simulink model "PubIfDecisionLM_MDL"  (R2020b)
settings: configuration reference "DspaceConfig" (kept outside this file)
PostLoadFcn:
  | if any(exist('dsrtsu_mdlpostloadfcn', 'file') ~= 0), dsrtsu_mdlpostloadfcn('Execute', bdroot); end
InitFcn:
  | , if any(exist('dsmpb_private', 'file') ~= 0), dsmpb_private('dsmpb_mdlclblib', 'Init', bdroot); end,
undefined symbols (not defined in the file or in its folder): OFM_OBJ_FUSIONTYPE_E, OFM_OBJ_MOVINGSTATE_E, OFM_OBJ_ORIENTATION_E, OFM_OBJ_TYPE_E, P_LM_Cyc, P_LM_EMLHistKapRcdBufSize, P_LM_EMLHistTrajBaseDis, P_LM_EMLHistTrajPNum, P_LM_EMLKapCorrMaxThre, P_LM_EMLMinKapThre, P_LM_EMLPathDisDiffThre, P_LM_EMLQuaFiltPar, P_LM_EMLTurnActKapThre, P_LM_EMLValidQuaThre, P_LM_FntPath1Disgap, P_LM_FntPath1MinDis, P_LM_FntPath1Timegap, P_LM_FntPath2Disgap, P_LM_FntPath2MinDis, P_LM_FntPath2Timegap, P_LM_FntPath3Disgap, P_LM_FntPath3MinDis, P_LM_FntPath3Timegap, P_LM_FusBLParFiltP, P_LM_FusEVDifC2Thre, P_LM_FusEVOPath1AllVSLDisThre, P_LM_FusEVOPath1AllVSLLostNumThre, P_LM_FusEVOPath1AllVSLQuaThre, P_LM_FusEVOPath1OTLFacNLC, P_LM_FusOTLQuaThre, P_LM_FusOTLSW, P_LM_FusParC0Index, P_LM_FusParC1Index, P_LM_FusParC2Index, P_LM_FusParC3Index, P_LM_FusVSLQuaThre, P_LM_FusVSLSW, P_LM_FusVSLValidSteerWheerAngThre, P_LM_FusVSLValidVxvThre, P_LM_LaneWidth, P_LM_OTLBufTPInfoEvaFactor, P_LM_OTLObjNum, P_LM_OTLObjSelectAgeThre, P_LM_OTLObjSelectDxAssessVx, P_LM_OTLObjSelectDxThre, P_LM_OTLObjSelectVxThre, P_LM_OTLObjSelectVyAssessDx, P_LM_OTLObjSelectVyThre, P_LM_OTLTrajPntBaseDis, P_LM_OTLTrajStdThre, P_LM_VSLAvailLineNum, P_LM_VSLBLSDiffThre, P_LM_VSLBLSDisRatio, P_LM_VSLFusBLParFiltP_C1, P_LM_VSLFusBLParFiltP_C2, P_LM_VSLFusBLParFiltP_C3, P_LM_VSLFusBLParFiltP_Quality, P_LM_VSLHistTrajBaseDis, P_LM_VSLHistTrajPNum, P_LM_VSLLCC0diff ... (+18)
libraries: simulink x145, LM_LIB x43
(part 1 of 24)
PreSaveFcn:
  | , if any(exist('dsmpb_private', 'file') ~= 0), dsmpb_private('dsmpb_mdlclblib', 'PreSave', bdroot); end,
CloseFcn:
  | , if any(exist('dsmpb_private', 'file') ~= 0), dsmpb_private('dsmpb_mdlclblib', 'Close', bdroot); end,
settings Model: DataDictionary=HWA_DDs.sldd  RTICANMMDATA=struct('GeneralSetupData',struct('modelroot','C:\Users\GW00133806\Desktop\ADAS_Store\Project\V61_Autobox_Noa\LM_TOS','generalsettings',struct('filesettings',struct('destfolder',struct('Name','RTICANMM_FILES','Check',1),'buildfolder',struct('Name','.','Check',1),'AbsDestfolder',struct('Name','C:\Users\GW00133806\Desktop\ADAS_Store\Project\V61_Autobox_Noa\LM_TOS\RTICANMM_FILES'),'AbsBuildfolder',struct('Name','C:\Users\GW00133806\Desktop\ADAS_Store\Project\V61_Autobox_Noa\LM_TOS'))),'options',struct('addpaths',1,'rmpaths',1,'addtrcexclusion',false,'cannavigator',struct('checkmonitoring',0),'show_usrtrc',0,'use_usrtrc',0),'advanced',struct('options',ones(1,100)),'MPSetup',{{}},'RTI',struct('Type','DSRT','Ver','4.2','Date','02-Nov-2019'),'modelname','PubIfDecisionLM_MDL','block','PubIfDecisionLM_MDL'))  DSRTSU_INTERNAL_RTIFPGA=150  Creator=GW00180895  LastModifiedBy=GW00133806
settings ConfigSetRef: SourceName=DspaceConfig

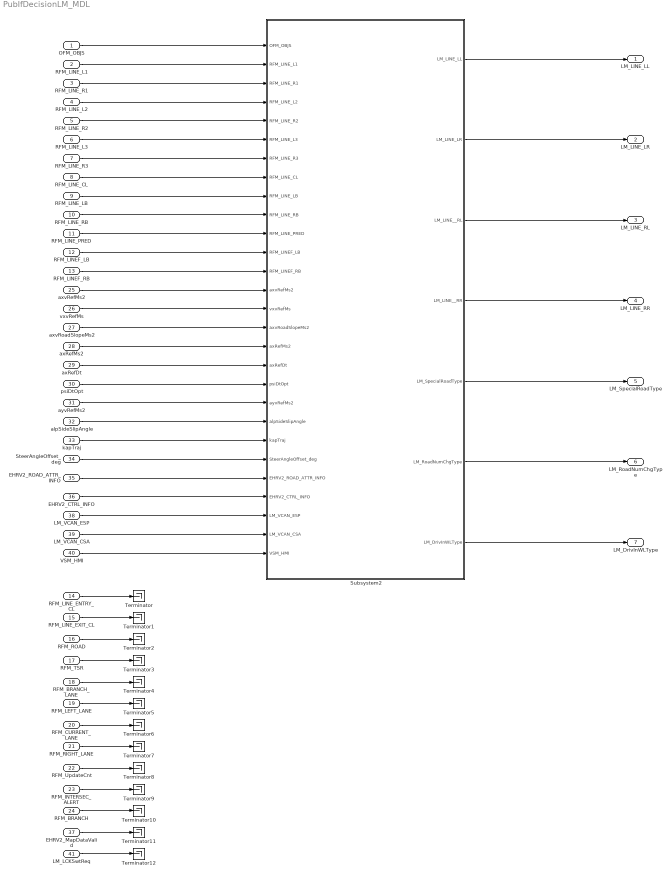
== system PubIfDecisionLM_MDL ==
  OFM_OBJS : Inport  OutDataTypeStr=Bus: OFM_OBJ_BUS  PortDimensions=1  BusOutputAsStruct=on
  RFM_LINE_L1 : Inport  Port=2  OutDataTypeStr=Bus: RFM_LINE_BUS  PortDimensions=1  BusOutputAsStruct=on
  RFM_LINE_R1 : Inport  Port=3  OutDataTypeStr=Bus: RFM_LINE_BUS  PortDimensions=1  BusOutputAsStruct=on
  RFM_LINE_L2 : Inport  Port=4  OutDataTypeStr=Bus: RFM_LINE_BUS  PortDimensions=1  BusOutputAsStruct=on
  RFM_LINE_R2 : Inport  Port=5  OutDataTypeStr=Bus: RFM_LINE_BUS  PortDimensions=1  BusOutputAsStruct=on
  RFM_LINE_L3 : Inport  Port=6  OutDataTypeStr=Bus: RFM_LINE_BUS  PortDimensions=1  BusOutputAsStruct=on
  RFM_LINE_R3 : Inport  Port=7  OutDataTypeStr=Bus: RFM_LINE_BUS  PortDimensions=1  BusOutputAsStruct=on
  RFM_LINE_CL : Inport  Port=8  OutDataTypeStr=Bus: RFM_LINE_BUS  PortDimensions=1  BusOutputAsStruct=on
  RFM_LINE_LB : Inport  Port=9  OutDataTypeStr=Bus: RFM_LINE_BUS  PortDimensions=1  BusOutputAsStruct=on
  RFM_LINE_RB : Inport  Port=10  OutDataTypeStr=Bus: RFM_LINE_BUS  PortDimensions=1  BusOutputAsStruct=on
  RFM_LINE_PRED : Inport  Port=11  OutDataTypeStr=Bus: RFM_LINE_BUS  PortDimensions=1  BusOutputAsStruct=on
  RFM_LINEF_LB : Inport  Port=12  OutDataTypeStr=Bus: RFM_LINE_BUS  PortDimensions=1  BusOutputAsStruct=on
  RFM_LINEF_RB : Inport  Port=13  OutDataTypeStr=Bus: RFM_LINE_BUS  PortDimensions=1  BusOutputAsStruct=on
  RFM_LINE_ENTRY_CL : Inport  Port=14  OutDataTypeStr=Bus: RFM_LINE_BUS  PortDimensions=1  BusOutputAsStruct=on
  RFM_LINE_EXIT_CL : Inport  Port=15  OutDataTypeStr=Bus: RFM_LINE_BUS  PortDimensions=1  BusOutputAsStruct=on
  RFM_ROAD : Inport  Port=16  OutDataTypeStr=Bus: RFM_ROAD_BUS  PortDimensions=1  BusOutputAsStruct=on
  RFM_TSR : Inport  Port=17  OutDataTypeStr=Bus: RFM_TSR_BUS  PortDimensions=1  BusOutputAsStruct=on
  RFM_BRANCH_LANE : Inport  Port=18  OutDataTypeStr=Bus: RFM_LANE_BUS  PortDimensions=1  BusOutputAsStruct=on
  RFM_LEFT_LANE : Inport  Port=19  OutDataTypeStr=Bus: RFM_LANE_BUS  PortDimensions=1  BusOutputAsStruct=on
  RFM_CURRENT_LANE : Inport  Port=20  OutDataTypeStr=Bus: RFM_LANE_BUS  PortDimensions=1  BusOutputAsStruct=on
  RFM_RIGHT_LANE : Inport  Port=21  OutDataTypeStr=Bus: RFM_LANE_BUS  PortDimensions=1  BusOutputAsStruct=on
  RFM_UpdateCnt : Inport  Port=22  OutDataTypeStr=uint32  PortDimensions=1  BusOutputAsStruct=on
  RFM_INTERSEC_ALERT : Inport  Port=23  OutDataTypeStr=Bus: RFM_INTERSEC_ALERT_BUS  PortDimensions=1  BusOutputAsStruct=on
  RFM_BRANCH : Inport  Port=24  OutDataTypeStr=Bus: RFM_BRANCH_BUS  PortDimensions=1  BusOutputAsStruct=on
  axvRefMs2 : Inport  Port=25  OutDataTypeStr=single  PortDimensions=1  BusOutputAsStruct=on
  vxvRefMs : Inport  Port=26  OutDataTypeStr=single  PortDimensions=1  BusOutputAsStruct=on
  axvRoadSlopeMs2 : Inport  Port=27  OutDataTypeStr=single  PortDimensions=1  BusOutputAsStruct=on
  axRefMs2 : Inport  Port=28  OutDataTypeStr=single  PortDimensions=1  BusOutputAsStruct=on
  axRefDt : Inport  Port=29  OutDataTypeStr=single  PortDimensions=1  BusOutputAsStruct=on
  psiDtOpt : Inport  Port=30  OutDataTypeStr=single  PortDimensions=1  BusOutputAsStruct=on
  ayvRefMs2 : Inport  Port=31  OutDataTypeStr=single  PortDimensions=1  BusOutputAsStruct=on
  alpSideSlipAngle : Inport  Port=32  OutDataTypeStr=single  PortDimensions=1  BusOutputAsStruct=on
  kapTraj : Inport  Port=33  OutDataTypeStr=single  PortDimensions=1  BusOutputAsStruct=on
  SteerAngleOffset_deg : Inport  Port=34  OutDataTypeStr=single  PortDimensions=1  BusOutputAsStruct=on
  EHRV2_ROAD_ATTR_INFO : Inport  Port=35  PortDimensions=1  BusOutputAsStruct=on
  EHRV2_CTRL_INFO : Inport  Port=36  PortDimensions=1  BusOutputAsStruct=on
  EHRV2_MapDataValid : Inport  Port=37  OutDataTypeStr=uint8  PortDimensions=1  BusOutputAsStruct=on
  LM_VCAN_ESP : Inport  Port=38  OutDataTypeStr=Bus: LM_VCAN_ESP_BUS  PortDimensions=1  BusOutputAsStruct=on
  LM_VCAN_CSA : Inport  Port=39  OutDataTypeStr=Bus: LM_VCAN_CSA_BUS  PortDimensions=1  BusOutputAsStruct=on
  VSM_HMI : Inport  Port=40  OutDataTypeStr=Bus: VSM_HMI_BUS  PortDimensions=1  BusOutputAsStruct=on
  LM_LCKSwtReq : Inport  Port=41  OutDataTypeStr=boolean  PortDimensions=1  BusOutputAsStruct=on
  Subsystem2 : Subsystem
  Terminator{,1..12} (13 alike) : Terminator
  LM_LINE_LL : Outport  OutDataTypeStr=Bus: LM_LINE_BUS  PortDimensions=1  BusOutputAsStruct=on
  LM_LINE_LR : Outport  Port=2  OutDataTypeStr=Bus: LM_LINE_BUS  PortDimensions=1  BusOutputAsStruct=on
  LM_LINE_RL : Outport  Port=3  OutDataTypeStr=Bus: LM_LINE_BUS  PortDimensions=1  BusOutputAsStruct=on
  LM_LINE_RR : Outport  Port=4  OutDataTypeStr=Bus: LM_LINE_BUS  PortDimensions=1  BusOutputAsStruct=on
  LM_SpecialRoadType : Outport  Port=5  OutDataTypeStr=uint8  PortDimensions=1  BusOutputAsStruct=on
  LM_RoadNumChgType : Outport  Port=6  OutDataTypeStr=uint8  PortDimensions=1  BusOutputAsStruct=on
  LM_DrivInWLType : Outport  Port=7  OutDataTypeStr=uint8  PortDimensions=1  BusOutputAsStruct=on
  wires:
  OFM_OBJS/1 -> Subsystem2/1(OFM_OBJS)
  RFM_LINE_L1/1 -> Subsystem2/2(RFM_LINE_L1)
  RFM_LINE_R1/1 -> Subsystem2/3(RFM_LINE_R1)
  RFM_LINE_L2/1 -> Subsystem2/4(RFM_LINE_L2)
  RFM_LINE_R2/1 -> Subsystem2/5(RFM_LINE_R2)
  RFM_LINE_L3/1 -> Subsystem2/6(RFM_LINE_L3)
  RFM_LINE_R3/1 -> Subsystem2/7(RFM_LINE_R3)
  RFM_LINE_CL/1 -> Subsystem2/8(RFM_LINE_CL)
  RFM_LINE_LB/1 -> Subsystem2/9(RFM_LINE_LB)
  RFM_LINE_RB/1 -> Subsystem2/10(RFM_LINE_RB)
  RFM_LINE_PRED/1 -> Subsystem2/11(RFM_LINE_PRED)
  RFM_LINEF_LB/1 -> Subsystem2/12(RFM_LINEF_LB)
  RFM_LINEF_RB/1 -> Subsystem2/13(RFM_LINEF_RB)
  axvRefMs2/1 -> Subsystem2/14(axvRefMs2)
  vxvRefMs/1 -> Subsystem2/15(vxvRefMs)
  axvRoadSlopeMs2/1 -> Subsystem2/16(axvRoadSlopeMs2)
  axRefMs2/1 -> Subsystem2/17(axRefMs2)
  axRefDt/1 -> Subsystem2/18(axRefDt)
  psiDtOpt/1 -> Subsystem2/19(psiDtOpt)
  ayvRefMs2/1 -> Subsystem2/20(ayvRefMs2)
  alpSideSlipAngle/1 -> Subsystem2/21(alpSideSlipAngle)
  kapTraj/1 -> Subsystem2/22(kapTraj)
  SteerAngleOffset_deg/1 -> Subsystem2/23(SteerAngleOffset_deg)
  EHRV2_ROAD_ATTR_INFO/1 -> Subsystem2/24(EHRV2_ROAD_ATTR_INFO)
  EHRV2_CTRL_INFO/1 -> Subsystem2/25(EHRV2_CTRL_INFO)
  LM_VCAN_ESP/1 -> Subsystem2/26(LM_VCAN_ESP)
  LM_VCAN_CSA/1 -> Subsystem2/27(LM_VCAN_CSA)
  VSM_HMI/1 -> Subsystem2/28(VSM_HMI)
  Subsystem2/1(LM_LINE_LL) -> LM_LINE_LL/1
  Subsystem2/2(LM_LINE_LR) -> LM_LINE_LR/1
  Subsystem2/3(LM_LINE__RL) -> LM_LINE_RL/1
  Subsystem2/4(LM_LINE__RR) -> LM_LINE_RR/1
  Subsystem2/5(LM_SpecialRoadType) -> LM_SpecialRoadType/1
  Subsystem2/6(LM_RoadNumChgType) -> LM_RoadNumChgType/1
  Subsystem2/7(LM_DrivInWLType) -> LM_DrivInWLType/1
  RFM_LINE_ENTRY_CL/1 -> Terminator/1
  RFM_LINE_EXIT_CL/1 -> Terminator1/1
  RFM_ROAD/1 -> Terminator2/1
  RFM_LEFT_LANE/1 -> Terminator5/1
  RFM_BRANCH_LANE/1 -> Terminator4/1
  RFM_TSR/1 -> Terminator3/1
  RFM_INTERSEC_ALERT/1 -> Terminator9/1
  RFM_BRANCH/1 -> Terminator10/1
  EHRV2_MapDataValid/1 -> Terminator11/1
  RFM_UpdateCnt/1 -> Terminator8/1
  RFM_RIGHT_LANE/1 -> Terminator7/1
  RFM_CURRENT_LANE/1 -> Terminator6/1
  LM_LCKSwtReq/1 -> Terminator12/1

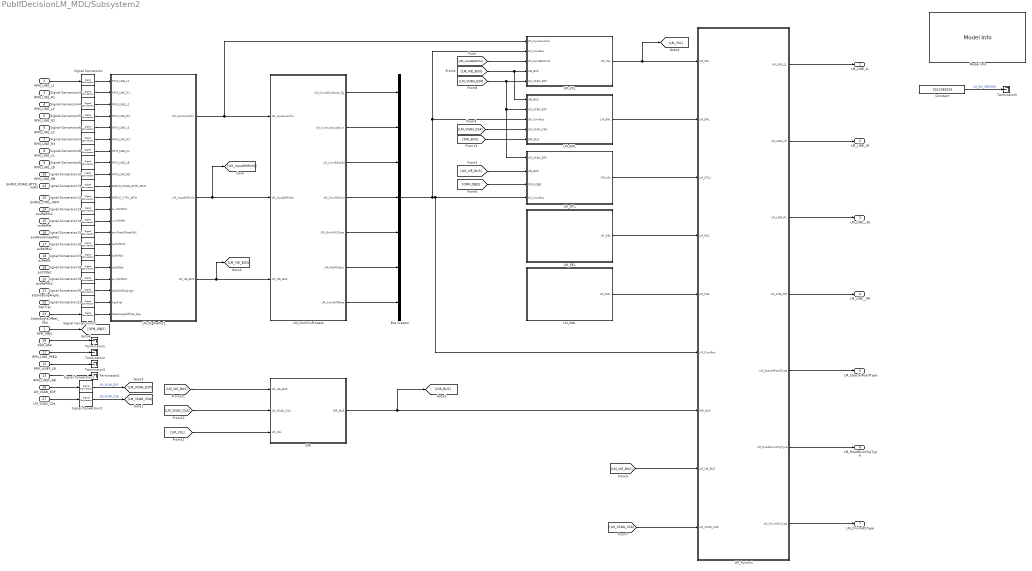
== system PubIfDecisionLM_MDL/Subsystem2 ==
  OFM_OBJS : Inport  OutDataTypeStr=Bus: OFM_OBJ_BUS  PortDimensions=1  BusOutputAsStruct=on
  RFM_LINE_L1 : Inport  Port=2  PortDimensions=1  BusOutputAsStruct=on
  RFM_LINE_R1 : Inport  Port=3  PortDimensions=1  BusOutputAsStruct=on
  RFM_LINE_L2 : Inport  Port=4  PortDimensions=1  BusOutputAsStruct=on
  RFM_LINE_R2 : Inport  Port=5  PortDimensions=1  BusOutputAsStruct=on
  RFM_LINE_L3 : Inport  Port=6  PortDimensions=1  BusOutputAsStruct=on
  RFM_LINE_R3 : Inport  Port=7  PortDimensions=1  BusOutputAsStruct=on
  RFM_LINE_CL : Inport  Port=8  PortDimensions=1  BusOutputAsStruct=on
  RFM_LINE_LB : Inport  Port=9  OutDataTypeStr=Bus: RFM_LINE_BUS  PortDimensions=1  BusOutputAsStruct=on
  RFM_LINE_RB : Inport  Port=10  OutDataTypeStr=Bus: RFM_LINE_BUS  PortDimensions=1  BusOutputAsStruct=on
  RFM_LINE_PRED : Inport  Port=11  OutDataTypeStr=Bus: RFM_LINE_BUS  PortDimensions=1  BusOutputAsStruct=on
  RFM_LINEF_LB : Inport  Port=12  OutDataTypeStr=Bus: RFM_LINE_BUS  PortDimensions=1  BusOutputAsStruct=on
  RFM_LINEF_RB : Inport  Port=13  OutDataTypeStr=Bus: RFM_LINE_BUS  PortDimensions=1  BusOutputAsStruct=on
  axvRefMs2 : Inport  Port=14  OutDataTypeStr=single  PortDimensions=1  BusOutputAsStruct=on
  vxvRefMs : Inport  Port=15  OutDataTypeStr=single  PortDimensions=1  BusOutputAsStruct=on
  axvRoadSlopeMs2 : Inport  Port=16  OutDataTypeStr=single  PortDimensions=1  BusOutputAsStruct=on
  axRefMs2 : Inport  Port=17  OutDataTypeStr=single  PortDimensions=1  BusOutputAsStruct=on
  axRefDt : Inport  Port=18  OutDataTypeStr=single  PortDimensions=1  BusOutputAsStruct=on
  psiDtOpt : Inport  Port=19  OutDataTypeStr=single  PortDimensions=1  BusOutputAsStruct=on
  ayvRefMs2 : Inport  Port=20  OutDataTypeStr=single  PortDimensions=1  BusOutputAsStruct=on
  alpSideSlipAngle : Inport  Port=21  OutDataTypeStr=single  PortDimensions=1  BusOutputAsStruct=on
  kapTraj : Inport  Port=22  OutDataTypeStr=single  PortDimensions=1  BusOutputAsStruct=on
  SteerAngleOffset_deg : Inport  Port=23  OutDataTypeStr=single  PortDimensions=1  BusOutputAsStruct=on
  EHRV2_ROAD_ATTR_INFO : Inport  Port=24  PortDimensions=1  BusOutputAsStruct=on
  EHRV2_CTRL_INFO : Inport  Port=25  PortDimensions=1  BusOutputAsStruct=on
  LM_VCAN_ESP : Inport  Port=26  OutDataTypeStr=Bus: LM_VCAN_ESP_BUS  PortDimensions=1  BusOutputAsStruct=on
  LM_VCAN_CSA : Inport  Port=27  OutDataTypeStr=Bus: LM_VCAN_CSA_BUS  PortDimensions=1  BusOutputAsStruct=on
  VSM_HMI : Inport  Port=28  OutDataTypeStr=Bus: VSM_HMI_BUS  PortDimensions=1  BusOutputAsStruct=on
  Bus Creator : BusCreator  Inputs=7
  Constant : Constant  Value=2012080301
  DIR : Subsystem
  LM_ComFcnProcess : Subsystem
  LM_EML : Subsystem
  LM_Fusion1 : Subsystem
  LM_MAL : Subsystem
  LM_OTL : Subsystem
  LM_REL : Subsystem
  LM_SigPrePro1 : Subsystem
  LM_VSL : Subsystem
  Model Info : simulink/Model-Wide Utilities/Model Info  Frame=on  DisplayStringWithTags=|  HorizontalTextAlignment=Left  LeftAlignmentValue=0.02
      | 2020/09/19
      | 当前支持功能：
      | 1.车道线清晰前方50m及后方80m道路模型
      | 2.无车道线情况前方max（30m，vxvref*2)及后方80m道路模型
      | 
      | 2020/09/30
      | 当前支持功能：
      | 1. 基于自车运动状态及基于摄像头的道路模型融合版本
      | 
      | 2020/10/1
      | 当前支持功能：
      | 1. 基于自车运动状态及基于摄像头的道路模型融合版本
      | 变更记录：
      | 1. 加入车道线C0自校验模块
      | 2. 针对两段轨迹分叉情况对应优化算法
      | 3. EHR车道数量模型内部给定默认值3
      | 4. L2&R2的有效距离融合内部给定100，会影响道路模型准确度，当前模型临时给定默认值30
      | 
      | 2020/10/14
      | 当前支持功能：
      | 1. 基于自车运动状态及基于摄像头的道路模型融合版本，可输出前方后方轨迹
      | 变更记录：
      | 1. 加入异常车道线剔除逻辑，避免异常车道线对道路模型的影响
      | 2. 适当延长车道线的道路模型的有效长度
      | 3. 优化VSL道路模型的基础质量计算
      | 
      | 2020/10/15
      | 当前支持功能：
      | 1. 基于自车运动状态及基于摄像头的道路模型融合版本，可输出前方后方轨迹
      | 变更记录：
      | 1. 优化VSL后方道路模型算法，增加对换道时车道线C0突变监控及组合选择后方轨迹点并拟合参数，提高了在换道过程中后方轨迹的稳定性
      | 2. 更改融合部分逻辑，当车道线清晰时，后方轨迹输出VSL道路模型
      | 
      | 2020/11/10
      | 变更记录：
      | 1.调节VSL中C0值的滤波系数0.15->0.65
      | 
      | 2020/11/17
      | 变更记录：
      | 1.增加OTL模块，并参与道路模型融合
      | 2.优化VSL后方轨迹逻辑
      | 
      | 2020/11/19
      | 变更记录：
      | 1.增加对道路模型输出结果是否为nan值的判断处理
      | 2.优化VSL后方轨迹逻辑算法
      | 
      | 2020/11/23
      | 变更记录：
      | 1.修复19号邻车道目标一直误选问题
      | 
      | 2020/11/27
      | 变更记录：
      | 1.优化VSL道路模型不准时的融合策略
      | 2.优化程序刚运行时的C0滤波策略
      | 3.更改监控车道线跳变部分bug
      | 4.优化EML和OTL融合策略
      | 5.优化VSL第2/3段轨迹放出和去除策略
      | 
      | 2020/12/03
      | 变更记录：
      | 1. 更新驾驶员模型模块逻辑
      | 2. 更新融合策略
      | 
      | 2020/12/08
      | 变更记录：
      | 1. 模型中添加观测变量
  Signal Conversion{,1..22} (23 alike) : SignalConversion  OverrideOpt=off
  Terminator{1..5} (5 alike) : Terminator
  LM_LINE_LL : Outport  OutDataTypeStr=Bus: LM_LINE_BUS  PortDimensions=1  BusOutputAsStruct=on
  LM_LINE_LR : Outport  Port=2  OutDataTypeStr=Bus: LM_LINE_BUS  PortDimensions=1  BusOutputAsStruct=on
  LM_LINE__RL : Outport  Port=3  OutDataTypeStr=Bus: LM_LINE_BUS  PortDimensions=1  BusOutputAsStruct=on
  LM_LINE__RR : Outport  Port=4  OutDataTypeStr=Bus: LM_LINE_BUS  PortDimensions=1  BusOutputAsStruct=on
  LM_SpecialRoadType : Outport  Port=5  OutDataTypeStr=uint8  PortDimensions=1  BusOutputAsStruct=on
  LM_RoadNumChgType : Outport  Port=6  OutDataTypeStr=uint8  PortDimensions=1  BusOutputAsStruct=on
  LM_DrivInWLType : Outport  Port=7  OutDataTypeStr=uint8  PortDimensions=1  BusOutputAsStruct=on
  wires:
  [LM_InputEHRInfo] -> LM_VSL/3(LM_InputEHRInfo)
  ayvRefMs2/1 -> Signal Conversion19/1
  LM_Fusion1/3(LM_LINE_RL) -> LM_LINE__RL/1
  [LM_VCAN_CSA] -> LM_EML/4(LM_VCAN_CSA)
  Signal Conversion2/1 -> [LM_VCAN_CSA]  "LM_VCAN_CSA"
  [LM_VIE_BUS] -> DIR/1(LM_VIE_BUS)
  RFM_LINE_L3/1 -> Signal Conversion6/1
  LM_Fusion1/5(LM_SpecialRoadType) -> LM_SpecialRoadType/1
  LM_Fusion1/6(LM_RoadNumChgType) -> LM_RoadNumChgType/1
  RFM_LINE_CL/1 -> Signal Conversion8/1
  LM_Fusion1/4(LM_LINE_RR) -> LM_LINE__RR/1
  VSM_HMI/1 -> Terminator1/1
  RFM_LINE_LB/1 -> Signal Conversion9/1
  psiDtOpt/1 -> Signal Conversion18/1
  [LM_VCAN_CSA] -> LM_Fusion1/9(LM_VCAN_CSA)
  LM_SigPrePro1/2(LM_InputEHRInfo) -> [LM_InputEHRInfo], LM_ComFcnProcess/2(LM_InputEHRInfo)
  [LM_VIE_BUS] -> LM_Fusion1/8(LM_VIE_BUS)
  RFM_LINE_R1/1 -> Signal Conversion3/1
  RFM_LINE_PRED/1 -> Terminator2/1
  LM_Fusion1/2(LM_LINE_LR) -> LM_LINE_LR/1
  LM_VSL/1(LM_VSL) -> [LM_VSL], LM_Fusion1/1(LM_VSL)
  kapTraj/1 -> Signal Conversion21/1
  alpSideSlipAngle/1 -> Signal Conversion20/1
  Constant/1 -> Terminator5/1  "LM_SW_VERSION"
  LM_ComFcnProcess/5(LM_DrivInWLType) -> Bus Creator/5
  axRefDt/1 -> Signal Conversion17/1
  LM_ComFcnProcess/7(LM_ComEVOffset) -> Bus Creator/7
  RFM_LINE_R2/1 -> Signal Conversion5/1
  axRefMs2/1 -> Signal Conversion16/1
  OFM_OBJS/1 -> [OFM_OBJS]
  SteerAngleOffset_deg/1 -> Signal Conversion22/1
  LM_ComFcnProcess/4(LM_ComRENum) -> Bus Creator/4
  RFM_LINE_L2/1 -> Signal Conversion4/1
  LM_ComFcnProcess/6(LM_PathDisBus) -> Bus Creator/6
  LM_MAL/1(LM_MAL) -> LM_Fusion1/5(LM_MAL)
  [DIR_BUS] -> LM_EML/5(DIR_BUS)
  RFM_LINEF_RB/1 -> Terminator4/1
  LM_ComFcnProcess/2(LM_ComLineLostNum) -> Bus Creator/2
  LM_EML/1(LM_EML) -> LM_Fusion1/2(LM_EML)
  DIR/1(DIR_BUS) -> [DIR_BUS], LM_Fusion1/7(DIR_BUS)
  RFM_LINE_L1/1 -> Signal Conversion/1
  [LM_VCAN_ESP] -> LM_VSL/5(LM_VCAN_ESP), LM_OTL/1(LM_VCAN_ESP), LM_EML/2(LM_VCAN_ESP)
  LM_Fusion1/7(LM_DrivInWLType) -> LM_DrivInWLType/1
  Bus Creator/1 -> LM_VSL/2(LM_ComBus), LM_EML/3(LM_ComBus), LM_OTL/4(LM_ComBus), LM_Fusion1/6(LM_ComBus)
  LM_OTL/1(OTLInfo) -> LM_Fusion1/3(LM_OTL1)
  vxvRefMs/1 -> Signal Conversion14/1
  RFM_LINE_RB/1 -> Signal Conversion10/1
  LM_SigPrePro1/3(LM_VIE_BUS) -> [LM_VIE_BUS], LM_ComFcnProcess/3(LM_VIE_BUS)
  LM_ComFcnProcess/3(LM_ComREValid) -> Bus Creator/3
  LM_REL/1(LM_REL) -> LM_Fusion1/4(LM_REL)
  LM_ComFcnProcess/1(LM_ComAllLineLost_flg) -> Bus Creator/1
  axvRoadSlopeMs2/1 -> Signal Conversion15/1
  [OFM_OBJS] -> LM_OTL/3(OFM_OBJS)
  Signal Conversion1/1 -> [LM_VCAN_ESP]  "LM_VCAN_ESP"
  axvRefMs2/1 -> Signal Conversion13/1
  EHRV2_ROAD_ATTR_INFO/1 -> Signal Conversion11/1
  RFM_LINEF_LB/1 -> Terminator3/1
  [LM_VSL] -> DIR/3(LM_VSL)
  LM_SigPrePro1/1(LM_InputLineInfo) -> LM_VSL/1(LM_InputLineInfo), LM_ComFcnProcess/1(LM_InputLineInfo)
  EHRV2_CTRL_INFO/1 -> Signal Conversion12/1
  RFM_LINE_R3/1 -> Signal Conversion7/1
  [LM_VIE_BUS] -> LM_VSL/4(VIE_BUS), LM_EML/1(VIE_BUS)
  [LM_VCAN_CSA] -> DIR/2(LM_VCAN_CSA)
  [LM_VIE_BUS] -> LM_OTL/2(VIE_BUS)
  LM_Fusion1/1(LM_LINE_LL) -> LM_LINE_LL/1
  LM_VCAN_CSA/1 -> Signal Conversion2/1
  LM_VCAN_ESP/1 -> Signal Conversion1/1
  Signal Conversion/1 -> LM_SigPrePro1/1(RFM_LINE_L1)
  Signal Conversion3/1 -> LM_SigPrePro1/2(RFM_LINE_R1)
  Signal Conversion4/1 -> LM_SigPrePro1/3(RFM_LINE_L2)
  Signal Conversion5/1 -> LM_SigPrePro1/4(RFM_LINE_R2)
  Signal Conversion7/1 -> LM_SigPrePro1/6(RFM_LINE_R3)
  Signal Conversion8/1 -> LM_SigPrePro1/7(RFM_LINE_CL)
  Signal Conversion9/1 -> LM_SigPrePro1/8(RFM_LINE_LB)
  Signal Conversion6/1 -> LM_SigPrePro1/5(RFM_LINE_L3)
  Signal Conversion11/1 -> LM_SigPrePro1/10(EHRV2_ROAD_ATTR_INFO)
  Signal Conversion12/1 -> LM_SigPrePro1/11(EHRV2_CTRL_INFO)
  Signal Conversion10/1 -> LM_SigPrePro1/9(RFM_LINE_RB)
  Signal Conversion16/1 -> LM_SigPrePro1/15(axRefMs2)
  Signal Conversion13/1 -> LM_SigPrePro1/12(axvRefMs2)
  Signal Conversion14/1 -> LM_SigPrePro1/13(vxvRefMs)
  Signal Conversion15/1 -> LM_SigPrePro1/14(axvRoadSlopeMs2)
  Signal Conversion17/1 -> LM_SigPrePro1/16(axRefDt)
  Signal Conversion20/1 -> LM_SigPrePro1/19(alpSideSlipAngle)
  Signal Conversion21/1 -> LM_SigPrePro1/20(kapTraj)
  Signal Conversion18/1 -> LM_SigPrePro1/17(psiDtOpt)
  Signal Conversion19/1 -> LM_SigPrePro1/18(ayvRefMs2)
  Signal Conversion22/1 -> LM_SigPrePro1/21(SteerAngleOffset_deg)

== system PubIfDecisionLM_MDL/Subsystem2/DIR ==
  LM_VIE_BUS : Inport
  LM_VCAN_CSA : Inport  Port=2
  LM_VSL : Inport  Port=3
  Bus Selector4 : BusSelector  OutputSignals=vxvRefMs,psiDtOpt,kapTraj
  Bus Selector5 : BusSelector  OutputSignals=SteerWheelAng,SteerWheelAngSign,LTurnLmpSwtSts,RTurnLmpSwtSts
  Bus Selector6 : BusSelector  OutputSignals=LM_VSLLRC0,LM_VSLRLC0,LM_VSLFntPath1P
  DrivingIntentionRecognition1 : Subsystem
  Selector : Selector  InputPortWidth=4  IndexOptions=Index vector (dialog)  Indices=3  OutputSizes=1
  DIR_BUS : Outport
  wires:
  Bus Selector4/3 -> DrivingIntentionRecognition1/3(kapTraj)  "<kapTraj>"
  Selector/1 -> DrivingIntentionRecognition1/10(LM_VSLFntPathBaseC1)
  Bus Selector6/2 -> DrivingIntentionRecognition1/9(LM_RLC0)  "<LM_VSLRLC0>"
  Bus Selector6/1 -> DrivingIntentionRecognition1/8(LM_LRC0)  "<LM_VSLLRC0>"
  Bus Selector5/1 -> DrivingIntentionRecognition1/4(SteerWheelAngle)  "<SteerWheelAng>"
  Bus Selector4/1 -> DrivingIntentionRecognition1/1(vxvRefMs)  "<vxvRefMs>"
  Bus Selector4/2 -> DrivingIntentionRecognition1/2(PsiDtOpt)  "<psiDtOpt>"
  Bus Selector5/2 -> DrivingIntentionRecognition1/5(SteerWheelAngleSign)  "<SteerWheelAngSign>"
  Bus Selector6/3 -> Selector/1  "<LM_VSLFntPath1P>"
  LM_VSL/1 -> Bus Selector6/1
  LM_VIE_BUS/1 -> Bus Selector4/1
  LM_VCAN_CSA/1 -> Bus Selector5/1
  DrivingIntentionRecognition1/1(DIR_BUS) -> DIR_BUS/1
  Bus Selector5/3 -> DrivingIntentionRecognition1/6(LeftTurnSWSts)  "<LTurnLmpSwtSts>"
  Bus Selector5/4 -> DrivingIntentionRecognition1/7(RightTurnSWSts)  "<RTurnLmpSwtSts>"

== system PubIfDecisionLM_MDL/Subsystem2/LM_ComFcnProcess ==
  LM_InputLineInfo : Inport
  LM_InputEHRInfo : Inport  Port=2
  LM_VIE_BUS : Inport  Port=3
  Bus Creator : BusCreator  Inputs=3
  Bus Selector : BusSelector  OutputSignals=LM_LINE_L1.bIsLineExist,LM_LINE_R1.bIsLineExist,LM_LINE_L2.bIsLineExist,LM_LINE_R2.bIsLineExist,LM_LINE_LB.bIsLineExist,LM_LINE_RB.bIsLineExist
  Bus Selector2 : BusSelector  OutputSignals=LM_LINE_L2.bIsLineExist,LM_LINE_L2.dC0V,LM_LINE_R2.bIsLineExist,LM_LINE_R2.dC0V,LM_LINE_L1.bIsLineExist,LM_LINE_L1.eLineType,LM_LINE_R1.bIsLineExist,LM_LINE_R1.eLineType,LM_LINE_LB.bIsLineExist,LM_LINE_LB.dC0V,LM_LINE_LB.dDisStart,LM_LINE_RB.bIsLineExist,LM_LINE_RB.dC0V,LM_LINE_RB.dDisStart
  Bus Selector5 : BusSelector  OutputSignals=psiDtOpt,vxvRefMs
  Constant : Constant  OutDataTypeStr=uint8
  Constant1 : Constant  Value=3  OutDataTypeStr=uint8
  Constant2 : Constant  Value=0  OutDataTypeStr=uint8
  Constant3 : Constant  Value=0  OutDataTypeStr=uint8
  LM_AllLineLostJudge : Subsystem
  LM_ComEVOffsetCalc : Subsystem
  LM_DisCalc4EachLine : Subsystem
  LM_DrivInWLJudge : Stateflow chart  TreatAsAtomicUnit=on
  Signal Conversion : SignalConversion  OverrideOpt=on
  Signal Conversion{1..19} (19 alike) : SignalConversion  OverrideOpt=off
  Switch : Switch  Criteria=u2 > Threshold
  Terminator : Terminator
  LM_ComAllLineLost_flg : Outport
  LM_ComLineLostNum : Outport  Port=2
  LM_ComREValid : Outport  Port=3
  LM_ComRENum : Outport  Port=4
  LM_DrivInWLType : Outport  Port=5
  LM_PathDisBus : Outport  Port=6
  LM_ComEVOffset : Outport  Port=7
  wires:
  LM_InputEHRInfo/1 -> Terminator/1
  Constant1/1 -> LM_DrivInWLJudge/15(NumOfLaneDrvDir)
  Constant/1 -> LM_DrivInWLJudge/16(DrivingOnHighWay)
  LM_DisCalc4EachLine/1(LM_PathDisBus) -> LM_PathDisBus/1
  LM_DrivInWLJudge/1(LM_DrivInWLType) -> Switch/1
  LM_AllLineLostJudge/4(LM_ComRENum) -> LM_ComRENum/1
  LM_AllLineLostJudge/3(LM_ComREValid) -> LM_ComREValid/1
  LM_AllLineLostJudge/2(LM_ComLineLostNum) -> LM_ComLineLostNum/1
  LM_AllLineLostJudge/1(LM_ComAllLineLost_flg) -> LM_ComAllLineLost_flg/1
  Signal Conversion7/1 -> LM_DrivInWLJudge/2(LM_L2dC0V)  "LM_L2dC0V"
  Signal Conversion6/1 -> LM_DrivInWLJudge/1(LM_L2bIsLineExist)  "LM_L2bIsLineExist"
  Signal Conversion5/1 -> LM_AllLineLostJudge/6(LM_RBbIsLineExist)  "LM_RBbIsLineExist"
  Signal Conversion4/1 -> LM_AllLineLostJudge/5(LM_LBbIsLineExist)  "LM_LBbIsLineExist"
  Signal Conversion3/1 -> LM_AllLineLostJudge/4(LM_R2bIsLineExist)  "LM_R2bIsLineExist"
  Signal Conversion2/1 -> LM_AllLineLostJudge/3(LM_L2bIsLineExist)  "LM_L2bIsLineExist"
  Signal Conversion1/1 -> LM_AllLineLostJudge/2(LM_R1bIsLineExist)  "LM_R1bIsLineExist"
  Signal Conversion/1 -> LM_AllLineLostJudge/1(LM_L1bIsLineExist)  "LM_L1bIsLineExist"
  Bus Selector/6 -> Signal Conversion5/1  "<bIsLineExist>"
  Bus Selector/5 -> Signal Conversion4/1  "<bIsLineExist>"
  Bus Selector/4 -> Signal Conversion3/1  "<bIsLineExist>"
  Bus Selector/3 -> Signal Conversion2/1  "<bIsLineExist>"
  Bus Selector/2 -> Signal Conversion1/1  "<bIsLineExist>"
  Bus Selector/1 -> Signal Conversion/1  "<bIsLineExist>"
  LM_InputLineInfo/1 -> Bus Selector/1, Bus Selector2/1
  Bus Selector2/1 -> Signal Conversion6/1  "<bIsLineExist>"
  Bus Selector2/2 -> Signal Conversion7/1  "<dC0V>"
  Bus Selector2/3 -> Signal Conversion8/1  "<bIsLineExist>"
  Bus Selector2/4 -> Signal Conversion9/1  "<dC0V>"
  Bus Selector2/5 -> Signal Conversion14/1  "<bIsLineExist>"
  Bus Selector2/6 -> Signal Conversion16/1  "<eLineType>"
  Bus Selector2/7 -> Signal Conversion15/1  "<bIsLineExist>"
  Bus Selector2/8 -> Signal Conversion17/1  "<eLineType>"
  LM_VIE_BUS/1 -> Bus Selector5/1
  Bus Selector5/2 -> LM_ComEVOffsetCalc/1(VxvRef_ms), LM_DisCalc4EachLine/1(LM_vxvRefMs), LM_DrivInWLJudge/18(vxvRefMs)  "<vxvRefMs>"
  Bus Selector5/1 -> LM_ComEVOffsetCalc/2(PsiDtOpt), LM_DrivInWLJudge/17(psiDtOpt)  "<psiDtOpt>"
  Signal Conversion8/1 -> LM_DrivInWLJudge/3(LM_R2bIsLineExist)  "LM_R2bIsLineExist"
  Signal Conversion9/1 -> LM_DrivInWLJudge/4(LM_R2dC0V)  "LM_R2dC0V"
  Signal Conversion14/1 -> LM_DrivInWLJudge/5(LM_L1bIsLineExist)  "LM_L1bIsLineExist"
  Signal Conversion16/1 -> LM_DrivInWLJudge/6(LM_L1eLineType)  "LM_L1eLineType"
  Signal Conversion15/1 -> LM_DrivInWLJudge/7(LM_R1bIsLineExist)  "LM_R1bIsLineExist"
  Signal Conversion17/1 -> LM_DrivInWLJudge/8(LM_R1eLineType)  "LM_R1eLineType"
  Signal Conversion10/1 -> LM_DrivInWLJudge/9(LM_LBbIsLineExist)  "LM_LBbIsLineExist"
  Signal Conversion11/1 -> LM_DrivInWLJudge/10(LM_LBdC0V)  "LM_LBdC0V"
  Signal Conversion12/1 -> LM_DrivInWLJudge/11(LM_LBdDisStart)  "LM_LBdDisStart"
  Signal Conversion13/1 -> LM_DrivInWLJudge/12(LM_RBbIsLineExist)  "LM_RBbIsLineExist"
  Bus Selector2/9 -> Signal Conversion10/1  "<bIsLineExist>"
  Bus Selector2/10 -> Signal Conversion11/1  "<dC0V>"
  Bus Selector2/11 -> Signal Conversion12/1  "<dDisStart>"
  Signal Conversion18/1 -> LM_DrivInWLJudge/13(LM_RBdC0V)  "LM_RBdC0V"
  Signal Conversion19/1 -> LM_DrivInWLJudge/14(LM_RBdDisStart)  "LM_RBdDisStart"
  Bus Selector2/14 -> Signal Conversion19/1  "<dDisStart>"
  Bus Selector2/13 -> Signal Conversion18/1  "<dC0V>"
  Bus Selector2/12 -> Signal Conversion13/1  "<bIsLineExist>"
  Switch/1 -> LM_DrivInWLType/1  "LM_DrivInWLType"
  Constant2/1 -> Switch/3
  Constant3/1 -> Switch/2
  LM_ComEVOffsetCalc/1(LM_ComEVOffsetX) -> Bus Creator/1
  LM_ComEVOffsetCalc/2(LM_ComEVOffsetY) -> Bus Creator/2
  LM_ComEVOffsetCalc/3(LM_ComEVOffsetAng) -> Bus Creator/3
  Bus Creator/1 -> LM_ComEVOffset/1

== system PubIfDecisionLM_MDL/Subsystem2/LM_EML ==
  VIE_BUS : Inport
  LM_VCAN_ESP : Inport  Port=2
  LM_ComBus : Inport  Port=3
  LM_VCAN_CSA : Inport  Port=4  OutDataTypeStr=Bus: LM_VCAN_CSA_BUS
  DIR_BUS : Inport  Port=5
  Bus Creator : BusCreator  Inputs=16
  Bus Selector : BusSelector  OutputSignals=kapTraj,vxvRefMs
  Bus Selector1 : BusSelector  OutputSignals=SteerWheelAng,SteerWheelSpd
  Bus Selector2 : BusSelector  OutputSignals=signal7.LM_ComEVOffsetX,signal7.LM_ComEVOffsetY,signal7.LM_ComEVOffsetAng,LM_PathDisBus.LM_RearPath1Dis,LM_PathDisBus.LM_RearPath2Dis,LM_PathDisBus.LM_RearPath3Dis
  Bus Selector3 : BusSelector  OutputSignals=LM_DrivInWLType
  Bus Selector4 : BusSelector  OutputSignals=LM_DIRTurnLeftValid,LM_DIRTurnRightValid
  Bus Selector5 : BusSelector  OutputSignals=VehStandstill
  Data Type Conversion1 : DataTypeConversion  OutDataTypeStr=single
  LM_EMLFntPath1 : Subsystem
  LM_EMLRearPath1 : Subsystem
  LM_EML : Outport
  wires:
  Bus Creator/1 -> LM_EML/1  "LM_EML"
  VIE_BUS/1 -> Bus Selector/1
  LM_VCAN_ESP/1 -> Bus Selector5/1
  Bus Selector/2 -> Data Type Conversion1/1  "<vxvRefMs>"
  LM_VCAN_CSA/1 -> Bus Selector1/1
  Bus Selector1/1 -> LM_EMLFntPath1/3(SteerWheelAngle)  "<SteerWheelAng>"
  Data Type Conversion1/1 -> LM_EMLRearPath1/1(VxvRef_ms), LM_EMLFntPath1/7(VxvRef_ms)
  Bus Selector2/4 -> LM_EMLRearPath1/5(LM_RearPath1Dis)  "<LM_RearPath1Dis>"
  LM_ComBus/1 -> Bus Selector2/1, Bus Selector3/1
  Bus Selector1/2 -> LM_EMLFntPath1/4(SteerWheelSpd)  "<SteerWheelSpd>"
  LM_EMLRearPath1/2(LM_EMLRearPath1Qulity) -> Bus Creator/12
  LM_EMLRearPath1/4(LM_EMLRearPath2Qulity) -> Bus Creator/14
  LM_EMLRearPath1/6(LM_EMLRearPath3Qulity) -> Bus Creator/16
  LM_EMLFntPath1/1(LM_EMLFntPath1P) -> Bus Creator/1
  LM_EMLFntPath1/2(LM_EMLFntPath1Quality) -> Bus Creator/2
  LM_EMLFntPath1/3(LM_EMLFntPath2P) -> Bus Creator/3
  LM_EMLFntPath1/4(LM_EMLFntPath2Quality) -> Bus Creator/4
  LM_EMLFntPath1/5(LM_EMLFntPath3P) -> Bus Creator/5
  LM_EMLFntPath1/6(LM_EMLFntPath3Quality) -> Bus Creator/6
  LM_EMLFntPath1/7(LM_EMLLLC0) -> Bus Creator/7
  LM_EMLFntPath1/8(LM_EMLLRC0) -> Bus Creator/8
  LM_EMLFntPath1/9(LM_EMLRLC0) -> Bus Creator/9
  LM_EMLFntPath1/10(LM_EMLRRC0) -> Bus Creator/10
  Bus Selector3/1 -> LM_EMLFntPath1/5(LM_DrivInWLType)  "<LM_DrivInWLType>"
  LM_EMLRearPath1/1(LM_EMLRearPath1P) -> Bus Creator/11
  LM_EMLRearPath1/3(LM_EMLRearPath2P) -> Bus Creator/13
  LM_EMLRearPath1/5(LM_EMLRearPath3P) -> Bus Creator/15
  Bus Selector/1 -> LM_EMLFntPath1/6(kapTraj)  "<kapTraj>"
  DIR_BUS/1 -> Bus Selector4/1
  Bus Selector4/1 -> LM_EMLFntPath1/1(DIR_TurnLeftValid)  "<LM_DIRTurnLeftValid>"
  Bus Selector4/2 -> LM_EMLFntPath1/2(DIR_TurnRightValid)  "<LM_DIRTurnRightValid>"
  Bus Selector5/1 -> LM_EMLRearPath1/8(VehStandstill)  "<VehStandstill>"
  Bus Selector2/5 -> LM_EMLRearPath1/6(LM_RearPath2Dis)  "<LM_RearPath2Dis>"
  Bus Selector2/6 -> LM_EMLRearPath1/7(LM_RearPath3Dis)  "<LM_RearPath3Dis>"
  Bus Selector2/1 -> LM_EMLRearPath1/2(LM_ComEVOffsetX)  "<LM_ComEVOffsetX>"
  Bus Selector2/2 -> LM_EMLRearPath1/3(LM_ComEVOffsetY)  "<LM_ComEVOffsetY>"
  Bus Selector2/3 -> LM_EMLRearPath1/4(LM_ComEVOffsetAng)  "<LM_ComEVOffsetAng>"

== system PubIfDecisionLM_MDL/Subsystem2/LM_Fusion1 ==
  LM_VSL : Inport
  LM_EML : Inport  Port=2
  LM_OTL1 : Inport  Port=3
  LM_REL : Inport  Port=4
  LM_MAL : Inport  Port=5
  LM_ComBus : Inport  Port=6
  DIR_BUS : Inport  Port=7
  LM_VIE_BUS : Inport  Port=8
  LM_VCAN_CSA : Inport  Port=9
  Bus Creator : BusCreator  Inputs=6  OutDataTypeStr=Bus: LM_FusBLInfoBus  NonVirtualBus=on
  Constant : Constant  Value=0  OutDataTypeStr=uint8
  Constant1 : Constant  Value=0  OutDataTypeStr=uint8
  Constant2 : Constant  Value=0  OutDataTypeStr=uint8
  LM_FusBaseLineFilt : Subsystem
  LM_FusBaseLineInfoCalc : Subsystem
  LM_FusLaneModelInfo : Subsystem
  LM_FusRatioCalc : Subsystem
  LM_Fus_BLConnectivityCheck : Subsystem
  LM_FusfCamValidInfoCalc : Subsystem
  Signal Conversion{,1..6} (7 alike) : SignalConversion  OverrideOpt=off
  LM_LINE_LL : Outport  OutDataTypeStr=Bus: LM_LINE_BUS  PortDimensions=1  BusOutputAsStruct=on
  LM_LINE_LR : Outport  Port=2  OutDataTypeStr=Bus: LM_LINE_BUS  PortDimensions=1  BusOutputAsStruct=on
  LM_LINE_RL : Outport  Port=3  OutDataTypeStr=Bus: LM_LINE_BUS  PortDimensions=1  BusOutputAsStruct=on
  LM_LINE_RR : Outport  Port=4  OutDataTypeStr=Bus: LM_LINE_BUS  PortDimensions=1  BusOutputAsStruct=on
  LM_SpecialRoadType : Outport  Port=5  OutDataTypeStr=uint8  PortDimensions=1  BusOutputAsStruct=on
  LM_RoadNumChgType : Outport  Port=6  OutDataTypeStr=uint8  PortDimensions=1  BusOutputAsStruct=on
  LM_DrivInWLType : Outport  Port=7  OutDataTypeStr=uint8  PortDimensions=1  BusOutputAsStruct=on
  wires:
  Constant/1 -> Signal Conversion4/1  "LM_SpecialRoadType"
  Constant1/1 -> Signal Conversion5/1  "LM_RoadNumChgType"
  LM_FusRatioCalc/2(LM_FusRatioInfo) -> LM_FusfCamValidInfoCalc/1(LM_FusRatioInfo), LM_FusBaseLineInfoCalc/1(LM_FusBLInfo)
  LM_MAL/1 -> LM_FusBaseLineInfoCalc/6(LM_MAL), LM_FusRatioCalc/5(LM_MAL)
  LM_REL/1 -> LM_FusBaseLineInfoCalc/5(LM_REL), LM_FusRatioCalc/4(LM_REL)
  LM_OTL1/1 -> LM_FusBaseLineInfoCalc/4(LM_OTL), LM_FusRatioCalc/3(LM_OTL1)
  LM_VSL/1 -> LM_FusBaseLineInfoCalc/2(LM_VSL), LM_FusRatioCalc/1(LM_VSL)
  LM_EML/1 -> LM_FusBaseLineInfoCalc/3(LM_EML), LM_FusRatioCalc/2(LM_EML)
  LM_ComBus/1 -> [LM_ComBus], LM_FusRatioCalc/6(LM_ComBus)
  LM_VIE_BUS/1 -> LM_FusRatioCalc/7(LM_VIE_BUS)
  Bus Creator/1 -> LM_FusBaseLineFilt/3(LM_FusBLInfo)  "LM_FusBLInfoBefFilt"
  LM_FusBaseLineInfoCalc/1(LM_FusBLFntPath1Info) -> Bus Creator/1
  LM_FusBaseLineInfoCalc/2(LM_FusBLFntPath2Info) -> Bus Creator/2
  LM_FusBaseLineInfoCalc/3(LM_FusBLFntPath3Info) -> Bus Creator/3
  LM_FusBaseLineInfoCalc/4(LM_FusBLRearPath1Info) -> Bus Creator/4
  LM_FusBaseLineInfoCalc/5(LM_FusBLRearPath2Info) -> Bus Creator/5
  LM_FusBaseLineInfoCalc/6(LM_FusBLRearPath3Info) -> Bus Creator/6
  LM_FusRatioCalc/1(LM_C0Info) -> LM_FusBaseLineFilt/2(LM_C0Info)
  LM_FusBaseLineFilt/2(LM_C0InfoFilt) -> LM_FusLaneModelInfo/2(LM_C0InfoFilt)
  [LM_ComBus] -> LM_FusLaneModelInfo/3(LM_ComBus)
  LM_FusLaneModelInfo/1(LM_LINE_LL) -> Signal Conversion/1
  LM_FusLaneModelInfo/2(LM_LINE_LR) -> Signal Conversion1/1
  LM_FusLaneModelInfo/3(LM_LINE_RL) -> Signal Conversion2/1
  LM_FusLaneModelInfo/4(LM_LINE_RR) -> Signal Conversion3/1
  DIR_BUS/1 -> [DIR_BUS], LM_FusRatioCalc/8(DIR_BUS)
  [DIR_BUS] -> LM_FusBaseLineFilt/1(DIR_BUS)
  LM_VCAN_CSA/1 -> LM_FusRatioCalc/9(LM_VCAN_CSA)
  LM_FusBaseLineFilt/1(LM_FusBLInfoFilt) -> LM_Fus_BLConnectivityCheck/2(LM_FusBLInfoFilt)
  LM_Fus_BLConnectivityCheck/1(LM_FusBLInfo) -> LM_FusLaneModelInfo/1(LM_FusBLInfoFilt)
  [LM_ComBus] -> LM_Fus_BLConnectivityCheck/1(LM_ComBus)
  LM_FusfCamValidInfoCalc/1(LM_FusfCamValidInfo) -> LM_FusLaneModelInfo/4(LM_FusfCamValidInfo)
  Constant2/1 -> Signal Conversion6/1  "LM_DrivInWLType"
  Signal Conversion/1 -> LM_LINE_LL/1
  Signal Conversion1/1 -> LM_LINE_LR/1
  Signal Conversion2/1 -> LM_LINE_RL/1
  Signal Conversion3/1 -> LM_LINE_RR/1
  Signal Conversion4/1 -> LM_SpecialRoadType/1
  Signal Conversion5/1 -> LM_RoadNumChgType/1
  Signal Conversion6/1 -> LM_DrivInWLType/1

== system PubIfDecisionLM_MDL/Subsystem2/LM_MAL ==
  Ground : Ground
  LM_MAL : Outport
  wires:
  Ground/1 -> LM_MAL/1  "LM_MAL"

== system PubIfDecisionLM_MDL/Subsystem2/LM_OTL ==
  LM_VCAN_ESP : Inport
  VIE_BUS : Inport  Port=2
  OFM_OBJS : Inport  Port=3  PortDimensions=1  BusOutputAsStruct=on
  LM_ComBus : Inport  Port=4
  LM_OTL_MovObjTrajFit : Subsystem
  LM_OTL_MovObjTrajRecord3 : Subsystem
  Unit Delay : UnitDelay  SampleTime=-1  HasFrameUpgradeWarning=on
  Unit Delay1 : UnitDelay  SampleTime=-1  HasFrameUpgradeWarning=on
  OTLInfo : Outport
  wires:
  Unit Delay1/1 -> LM_OTL_MovObjTrajRecord3/2(LM_OTLBufTPInfoBusK1)
  Unit Delay/1 -> LM_OTL_MovObjTrajRecord3/1(LM_OTLBufTPVectBusK1)
  LM_OTL_MovObjTrajRecord3/1(LM_OTLBufTPVectBus) -> Unit Delay/1, LM_OTL_MovObjTrajFit/1(LM_OTLBufTPVectBus)
  OFM_OBJS/1 -> LM_OTL_MovObjTrajRecord3/5(OFM_OBJS)
  VIE_BUS/1 -> LM_OTL_MovObjTrajRecord3/4(VIE_BUS)
  LM_VCAN_ESP/1 -> LM_OTL_MovObjTrajRecord3/3(LM_VCAN_ESP)
  LM_ComBus/1 -> LM_OTL_MovObjTrajRecord3/6(LM_ComBus), LM_OTL_MovObjTrajFit/3(LM_ComBus)
  LM_OTL_MovObjTrajRecord3/2(LM_OTLBufTPInfoBus) -> Unit Delay1/1, LM_OTL_MovObjTrajFit/2(LM_OTLBufTPInfoBus)
  LM_OTL_MovObjTrajFit/1(OTLInfo) -> OTLInfo/1

== system PubIfDecisionLM_MDL/Subsystem2/LM_REL ==
  Ground : Ground
  LM_REL : Outport
  wires:
  Ground/1 -> LM_REL/1  "LM_REL"

== system PubIfDecisionLM_MDL/Subsystem2/LM_SigPrePro1 ==
  RFM_LINE_L1 : Inport
  RFM_LINE_R1 : Inport  Port=2
  RFM_LINE_L2 : Inport  Port=3
  RFM_LINE_R2 : Inport  Port=4
  RFM_LINE_L3 : Inport  Port=5
  RFM_LINE_R3 : Inport  Port=6
  RFM_LINE_CL : Inport  Port=7
  RFM_LINE_LB : Inport  Port=8
  RFM_LINE_RB : Inport  Port=9
  EHRV2_ROAD_ATTR_INFO : Inport  Port=10
  EHRV2_CTRL_INFO : Inport  Port=11
  axvRefMs2 : Inport  Port=12  OutDataTypeStr=single  PortDimensions=1  BusOutputAsStruct=on
  vxvRefMs : Inport  Port=13  OutDataTypeStr=single  PortDimensions=1  BusOutputAsStruct=on
  axvRoadSlopeMs2 : Inport  Port=14  OutDataTypeStr=single  PortDimensions=1  BusOutputAsStruct=on
  axRefMs2 : Inport  Port=15  OutDataTypeStr=single  PortDimensions=1  BusOutputAsStruct=on
  axRefDt : Inport  Port=16  OutDataTypeStr=single  PortDimensions=1  BusOutputAsStruct=on
  psiDtOpt : Inport  Port=17  OutDataTypeStr=single  PortDimensions=1  BusOutputAsStruct=on
  ayvRefMs2 : Inport  Port=18  OutDataTypeStr=single  PortDimensions=1  BusOutputAsStruct=on
  alpSideSlipAngle : Inport  Port=19  OutDataTypeStr=single  PortDimensions=1  BusOutputAsStruct=on
  kapTraj : Inport  Port=20  OutDataTypeStr=single  PortDimensions=1  BusOutputAsStruct=on
  SteerAngleOffset_deg : Inport  Port=21  OutDataTypeStr=single  PortDimensions=1  BusOutputAsStruct=on
  Bus Creator : BusCreator  Inputs=10
  Bus Creator1 : BusCreator  Inputs=2
  Signal Conversion{,1..9} (10 alike) : SignalConversion  OverrideOpt=off
  Subsystem1 : Subsystem
  LM_InputLineInfo : Outport
  LM_InputEHRInfo : Outport  Port=2
  LM_VIE_BUS : Outport  Port=3
  wires:
  SteerAngleOffset_deg/1 -> Signal Conversion9/1  "LM_SteerAngleOffset_deg"
  kapTraj/1 -> Signal Conversion8/1  "LM_kapTraj"
  alpSideSlipAngle/1 -> Signal Conversion7/1  "LM_alpSideSlipAngle"
  ayvRefMs2/1 -> Signal Conversion6/1  "LM_ayvRefMs2"
  psiDtOpt/1 -> Signal Conversion5/1  "LM_psiDtOpt"
  axRefDt/1 -> Signal Conversion4/1  "LM_axRefDt"
  axRefMs2/1 -> Signal Conversion3/1  "LM_axRefMs2"
  axvRoadSlopeMs2/1 -> Signal Conversion2/1  "LM_axvRoadSlopeMs2"
  vxvRefMs/1 -> Signal Conversion1/1  "LM_vxvRefMs"
  axvRefMs2/1 -> Signal Conversion/1  "LM_axvRefMs2"
  EHRV2_ROAD_ATTR_INFO/1 -> Bus Creator1/1  "EHRV2_ROAD_ATTR_INFO"
  EHRV2_CTRL_INFO/1 -> Bus Creator1/2  "EHRV2_CTRL_INFO"
  Bus Creator1/1 -> LM_InputEHRInfo/1  "LM_InputEHRInfo"
  Bus Creator/1 -> LM_VIE_BUS/1  "LM_VIE_BUS"
  RFM_LINE_L1/1 -> Subsystem1/1(RFM_LINE_L1_k)  "LM_RFM_LINE_L1"
  RFM_LINE_R1/1 -> Subsystem1/2(RFM_LINE_R1_k)  "LM_RFM_LINE_R1"
  RFM_LINE_L2/1 -> Subsystem1/3(RFM_LINE_L2_k)  "LM_RFM_LINE_L2"
  RFM_LINE_R2/1 -> Subsystem1/4(RFM_LINE_R2_k)  "LM_RFM_LINE_R2"
  RFM_LINE_L3/1 -> Subsystem1/5(RFM_LINE_L3_k)
  RFM_LINE_R3/1 -> Subsystem1/6(RFM_LINE_R3_k)
  RFM_LINE_CL/1 -> Subsystem1/7(RFM_LINE_CL_k)  "LM_RFM_LINE_CL"
  RFM_LINE_LB/1 -> Subsystem1/8(RFM_LINE_LB_k)  "LM_RFM_LINE_LB"
  RFM_LINE_RB/1 -> Subsystem1/9(RFM_LINE_RB_k)  "LM_RFM_LINE_RB"
  Subsystem1/1(LM_InputLineInfo) -> LM_InputLineInfo/1
  Signal Conversion/1 -> Bus Creator/1  "axvRefMs2"
  Signal Conversion1/1 -> Bus Creator/2  "vxvRefMs"
  Signal Conversion2/1 -> Bus Creator/3  "axvRoadSlopeMs2"
  Signal Conversion3/1 -> Bus Creator/4  "axRefMs2"
  Signal Conversion4/1 -> Bus Creator/5  "axRefDt"
  Signal Conversion5/1 -> Bus Creator/6  "psiDtOpt"
  Signal Conversion6/1 -> Bus Creator/7  "ayvRefMs2"
  Signal Conversion7/1 -> Bus Creator/8  "alpSideSlipAngle"
  Signal Conversion8/1 -> Bus Creator/9  "kapTraj"
  Signal Conversion9/1 -> Bus Creator/10  "SteerAngleOffset_deg"

== system PubIfDecisionLM_MDL/Subsystem2/LM_VSL ==
  LM_InputLineInfo : Inport
  LM_ComBus : Inport  Port=2
  LM_InputEHRInfo : Inport  Port=3
  VIE_BUS : Inport  Port=4
  LM_VCAN_ESP : Inport  Port=5
  Bus Creator1 : BusCreator  Inputs=17
  Bus Selector1 : BusSelector  OutputSignals=RFM_LINE
  LM_VSLFntPath : Subsystem
  LM_VSLRearPath : Subsystem
  LM_VSL : Outport
  wires:
  Bus Selector1/1 -> LM_VSLRearPath/3(RFM_LINE)  "<RFM_LINE>"
  Bus Creator1/1 -> LM_VSL/1  "LM_VSL"
  LM_ComBus/1 -> LM_VSLFntPath/2(LM_ComBus), LM_VSLRearPath/2(LM_ComBus)
  VIE_BUS/1 -> LM_VSLRearPath/4(VIE_BUS)
  LM_InputLineInfo/1 -> Bus Selector1/1, LM_VSLFntPath/1(LM_InputLineInfo)
  LM_VSLFntPath/1(LM_VSLFntPath1P) -> Bus Creator1/1, LM_VSLRearPath/1(LM_VSLFntPath1P)
  LM_VSLFntPath/2(LM_VSLFntPath1Quality) -> Bus Creator1/2
  LM_VSLFntPath/3(LM_VSLFntPath2P) -> Bus Creator1/3
  LM_VSLFntPath/4(LM_VSLFntPath2Quality) -> Bus Creator1/4
  LM_VSLFntPath/5(LM_VSLFntPath3P) -> Bus Creator1/5
  LM_VSLFntPath/6(LM_VSLFntPath3Quality) -> Bus Creator1/6
  LM_VSLRearPath/1(LM_VSLRearPath1P) -> Bus Creator1/12
  LM_VSLRearPath/2(LM_VSLRearPath1Qulity) -> Bus Creator1/13
  LM_VSLRearPath/3(LM_VSLRearPath2P) -> Bus Creator1/14
  LM_VSLRearPath/4(LM_VSLRearPath2Qulity) -> Bus Creator1/15
  LM_VSLRearPath/5(LM_VSLRearPath3P) -> Bus Creator1/16
  LM_VSLRearPath/6(LM_VSLRearPath3Qulity) -> Bus Creator1/17
  LM_VSLFntPath/7(LM_VSLBaseDis) -> Bus Creator1/7
  LM_InputEHRInfo/1 -> LM_VSLFntPath/3(LM_InputEHRInfo)
  LM_VSLFntPath/8(LM_VSLLLC0) -> Bus Creator1/8
  LM_VSLFntPath/9(LM_VSLLRC0) -> Bus Creator1/9
  LM_VSLFntPath/10(LM_VSLRLC0) -> Bus Creator1/10
  LM_VSLFntPath/11(LM_VSLRRC0) -> Bus Creator1/11
  LM_VCAN_ESP/1 -> LM_VSLRearPath/5(LM_VCAN_ESP)

== system PubIfDecisionLM_MDL/Subsystem2/DIR/DrivingIntentionRecognition1 ==
  vxvRefMs : Inport
  PsiDtOpt : Inport  Port=2
  kapTraj : Inport  Port=3
  SteerWheelAngle : Inport  Port=4
  SteerWheelAngleSign : Inport  Port=5
  LeftTurnSWSts : Inport  Port=6
  RightTurnSWSts : Inport  Port=7
  LM_LRC0 : Inport  Port=8
  LM_RLC0 : Inport  Port=9
  LM_VSLFntPathBaseC1 : Inport  Port=10
  Bus Creator : BusCreator  Inputs=4
  DIR_LaneChangeProbCalc : Subsystem
  DIR_TurnDirProbCalc : Subsystem
  DIR_TurnLampTimeCalc : Subsystem
  DIR_BUS : Outport
  wires:
  LM_RLC0/1 -> DIR_LaneChangeProbCalc/9(LM_RLC0)
  LM_LRC0/1 -> DIR_LaneChangeProbCalc/8(LM_LRC0)
  RightTurnSWSts/1 -> DIR_TurnDirProbCalc/7(RightTurnSWSts), DIR_TurnLampTimeCalc/2(RightTurnSWSts), DIR_LaneChangeProbCalc/3(RightTurnSWSts)
  LeftTurnSWSts/1 -> DIR_TurnDirProbCalc/6(LeftTurnSWSts), DIR_TurnLampTimeCalc/1(LeftTurnSWSts), DIR_LaneChangeProbCalc/4(LeftTurnSWSts)
  LM_VSLFntPathBaseC1/1 -> DIR_LaneChangeProbCalc/10(LM_VSLFntPathBaseC1)
  Bus Creator/1 -> DIR_BUS/1
  DIR_LaneChangeProbCalc/2(DIR_LC2RigProb) -> Bus Creator/4
  DIR_TurnDirProbCalc/2(DIR_TurnRightProb) -> Bus Creator/2
  DIR_TurnDirProbCalc/1(DIR_TurnLeftProb) -> Bus Creator/1
  DIR_LaneChangeProbCalc/1(DIR_LC2LeProb) -> Bus Creator/3
  DIR_TurnLampTimeCalc/1(DIR_LeftTurnLampOnTime) -> DIR_TurnDirProbCalc/8(DIR_LeftTurnLampOnTime), DIR_LaneChangeProbCalc/2(DIR_LeftTurnLampOnTime)
  DIR_TurnLampTimeCalc/2(DIR_RightTurnLampOnTime) -> DIR_TurnDirProbCalc/9(DIR_RightTurnLampOnTime), DIR_LaneChangeProbCalc/1(DIR_RightTurnLampOnTime)
  PsiDtOpt/1 -> DIR_TurnDirProbCalc/1(PsiDtOpt)
  vxvRefMs/1 -> DIR_LaneChangeProbCalc/7(vxvRefMs), DIR_TurnDirProbCalc/3(vxvRefMs)
  kapTraj/1 -> DIR_TurnDirProbCalc/2(kapTraj)
  SteerWheelAngle/1 -> DIR_LaneChangeProbCalc/6(SteerWheelAngle), DIR_TurnDirProbCalc/4(SteerWheelAngle)
  SteerWheelAngleSign/1 -> DIR_LaneChangeProbCalc/5(SteerWheelAngleSign), DIR_TurnDirProbCalc/5(SteerWheelAngleSign)

== system PubIfDecisionLM_MDL/Subsystem2/LM_ComFcnProcess/LM_AllLineLostJudge ==
  LM_L1bIsLineExist : Inport
  LM_R1bIsLineExist : Inport  Port=2
  LM_L2bIsLineExist : Inport  Port=3
  LM_R2bIsLineExist : Inport  Port=4
  LM_LBbIsLineExist : Inport  Port=5
  LM_RBbIsLineExist : Inport  Port=6
  Add : Sum  Inputs=++++
  Add1 : Sum
  Constant : Constant  OutDataTypeStr=uint8
  Constant1 : Constant  OutDataTypeStr=uint8
  Constant2 : Constant  Value=0  OutDataTypeStr=uint8
  Constant3 : Constant  Value=2  OutDataTypeStr=uint8
  Constant4 : Constant  OutDataTypeStr=uint8
  Constant5 : Constant  Value=0  OutDataTypeStr=uint8
  Logical Operator : Logic  Inputs=4  AllPortsSameDT=off  OutDataTypeStr=boolean
  Logical Operator1 : Logic  Operator=OR  AllPortsSameDT=off  OutDataTypeStr=boolean
  Relational Operator{,1..5} (6 alike) : RelationalOperator  Operator===  OutDataTypeStr=boolean  RndMeth=Nearest
  Switch{,1..5} (6 alike) : Switch  Criteria=u2 ~= 0
  LM_ComAllLineLost_flg : Outport
  LM_ComLineLostNum : Outport  Port=2
  LM_ComREValid : Outport  Port=3
  LM_ComRENum : Outport  Port=4
  wires:
  Add1/1 -> LM_ComRENum/1  "LM_ComRENum"
  Switch5/1 -> Add1/2
  Switch4/1 -> Add1/1
  Constant5/1 -> Switch4/3, Switch5/3
  Constant4/1 -> Switch5/1, Switch4/1
  Logical Operator1/1 -> LM_ComREValid/1  "LM_ComREValid"
  Relational Operator5/1 -> Logical Operator1/2, Switch5/2
  Relational Operator4/1 -> Logical Operator1/1, Switch4/2
  Constant3/1 -> Relational Operator4/2, Relational Operator5/2
  LM_RBbIsLineExist/1 -> Relational Operator5/1
  LM_LBbIsLineExist/1 -> Relational Operator4/1
  Add/1 -> LM_ComLineLostNum/1  "LM_ComLineLostNum"
  Switch3/1 -> Add/4
  Switch2/1 -> Add/3
  Switch1/1 -> Add/2
  Switch/1 -> Add/1
  Constant2/1 -> Switch1/3, Switch2/3, Switch3/3, Switch/3
  Constant1/1 -> Switch/1, Switch1/1, Switch2/1, Switch3/1
  Logical Operator/1 -> LM_ComAllLineLost_flg/1  "LM_ComAllLineLost_flg"
  Relational Operator3/1 -> Logical Operator/4, Switch3/2
  Relational Operator2/1 -> Logical Operator/3, Switch2/2
  Relational Operator1/1 -> Logical Operator/2, Switch1/2
  LM_R2bIsLineExist/1 -> Relational Operator3/1
  LM_L2bIsLineExist/1 -> Relational Operator2/1
  LM_R1bIsLineExist/1 -> Relational Operator1/1
  Relational Operator/1 -> Logical Operator/1, Switch/2
  Constant/1 -> Relational Operator1/2, Relational Operator2/2, Relational Operator3/2, Relational Operator/2
  LM_L1bIsLineExist/1 -> Relational Operator/1

== system PubIfDecisionLM_MDL/Subsystem2/LM_ComFcnProcess/LM_ComEVOffsetCalc ==
  note: rcs-reference coordinate system
  VxvRef_ms : Inport
  PsiDtOpt : Inport  Port=2
  Abs : Abs
  Constant : Constant  Value=0
  Constant1 : Constant  Value=0
  Constant2 : Constant  Value=0
  Constant3 : Constant  Value=0  OutDataTypeStr=single
  Constant4 : Constant  Value=P_LM_Cyc
  Constant5 : Constant  OutDataTypeStr=single
  Constant6 : Constant  Value=P_LM_Cyc
  Constant7 : Constant  Value=0  OutDataTypeStr=boolean
  Divide : Product  Inputs=*/
  DocBlock : simulink/Model-Wide Utilities/DocBlock  DocumentType=Text
      content=|
      | ## author:
      | livie
      | ## Data:
      | Nov 5,2019
      | ## Description:
      | calculate the offset of vehicle coordinate system in x、y、z direction
  Gain : Gain  Gain=-1
  Math Function1 : Math  Operator=square  SignedPower=on  SaturateOnIntegerOverflow=on
  Product{,1..4} (5 alike) : Product
  Relational Operator : RelationalOperator  Operator=<=  OutDataTypeStr=boolean  RndMeth=Nearest
  Relational Operator1 : RelationalOperator  Operator===  OutDataTypeStr=boolean  RndMeth=Nearest
  Subtract : Sum  Inputs=+-
  Switch{,1..3} (4 alike) : Switch  Criteria=u2 ~= 0
  Trigonometric Function : Trigonometry  Operator=cos
  Trigonometric Function1 : Trigonometry
  LM_ComEVOffsetX : Outport
  LM_ComEVOffsetY : Outport  Port=2
  LM_ComEVOffsetAng : Outport  Port=3
  wires:
  Abs/1 -> Relational Operator/1, Switch/3
  Product4/1 -> Switch3/3
  Trigonometric Function1/1 -> Product4/2
  Product3/1 -> Switch3/1
  Constant6/1 -> Product3/2
  Product2/1 -> Switch2/3
  Trigonometric Function/1 -> Subtract/2
  Constant5/1 -> Subtract/1
  Subtract/1 -> Product2/2
  Divide/1 -> Product2/1, Product4/1  "R"
  Switch3/1 -> LM_ComEVOffsetX/1  "LM_ComEVOffsetX"
  Switch2/1 -> LM_ComEVOffsetY/1  "LM_ComEVOffsetY"
  Product1/1 -> Switch1/3, Trigonometric Function/1, Trigonometric Function1/1
  Constant4/1 -> Product1/2
  Constant3/1 -> Switch2/1, Switch1/1
  Gain/1 -> LM_ComEVOffsetAng/1  "LM_ComEVOffsetAng"
  Constant7/1 -> Switch1/2, Switch2/2, Switch3/2
  Constant2/1 -> Relational Operator1/2
  Switch/1 -> Relational Operator1/1
  Constant1/1 -> Switch/1
  Relational Operator/1 -> Switch/2
  Constant/1 -> Relational Operator/2
  Product/1 -> Divide/2  "ay"
  Math Function1/1 -> Divide/1
  VxvRef_ms/1 -> Math Function1/1, Product/1, Product3/1
  PsiDtOpt/1 -> Product/2, Abs/1, Product1/1
  Switch1/1 -> Gain/1

== system PubIfDecisionLM_MDL/Subsystem2/LM_ComFcnProcess/LM_DisCalc4EachLine ==
  LM_vxvRefMs : Inport
  Bus Creator : BusCreator  Inputs=8
  LM_FrontDisCalc : Subsystem
  LM_RearDisCalc : Subsystem
  LM_PathDisBus : Outport
  wires:
  Bus Creator/1 -> LM_PathDisBus/1  "LM_PathDisBus"
  LM_RearDisCalc/3(LM_RearPath3Dis) -> Bus Creator/8  "LM_RearPath3Dis"
  LM_RearDisCalc/2(LM_RearPath2Dis) -> Bus Creator/7  "LM_RearPath2Dis"
  LM_RearDisCalc/1(LM_RearPath1Dis) -> Bus Creator/6  "LM_RearPath1Dis"
  LM_FrontDisCalc/5(LM_FntPath5Dis) -> Bus Creator/5
  LM_FrontDisCalc/4(LM_FntPath4Dis) -> Bus Creator/4
  LM_FrontDisCalc/3(LM_FntPath3Dis) -> Bus Creator/3  "LM_FntPath3Dis"
  LM_FrontDisCalc/2(LM_FntPath2Dis) -> Bus Creator/2  "LM_FntPath2Dis"
  LM_FrontDisCalc/1(LM_FntPath1Dis) -> Bus Creator/1  "LM_FntPath1Dis"
  LM_vxvRefMs/1 -> LM_FrontDisCalc/1(LM_vxvRefMs)

== system PubIfDecisionLM_MDL/Subsystem2/LM_EML/LM_EMLFntPath1 ==
  DIR_TurnLeftValid : Inport
  DIR_TurnRightValid : Inport  Port=2
  SteerWheelAngle : Inport  Port=3
  SteerWheelSpd : Inport  Port=4
  LM_DrivInWLType : Inport  Port=5
  kapTraj : Inport  Port=6
  VxvRef_ms : Inport  Port=7
  LM_EMLFntPathParCalc : Subsystem
  LM_EMLFntPathQualityCalc : Subsystem
  LM_EMLKapAdjVal : Subsystem
  LM_EML_C0 : Subsystem
  LM_EMLFntPath1P : Outport
  LM_EMLFntPath1Quality : Outport  Port=2
  LM_EMLFntPath2P : Outport  Port=3
  LM_EMLFntPath2Quality : Outport  Port=4
  LM_EMLFntPath3P : Outport  Port=5
  LM_EMLFntPath3Quality : Outport  Port=6
  LM_EMLLLC0 : Outport  Port=7
  LM_EMLLRC0 : Outport  Port=8
  LM_EMLRLC0 : Outport  Port=9
  LM_EMLRRC0 : Outport  Port=10
  wires:
  SteerWheelAngle/1 -> LM_EMLFntPathQualityCalc/2(SteerWheelAngle)
  VxvRef_ms/1 -> LM_EMLFntPathQualityCalc/1(VxvRef_ms)
  LM_EMLKapAdjVal/1(LM_EMLKap) -> LM_EMLFntPathParCalc/1(LM_EMLFntPathkap)
  SteerWheelSpd/1 -> LM_EMLFntPathQualityCalc/3(SteerWheelSpd)
  LM_EMLFntPathQualityCalc/1(LM_EMLFntPath1Quality) -> LM_EMLFntPath1Quality/1
  LM_EMLFntPathQualityCalc/2(LM_EMLFntPath2Quality) -> LM_EMLFntPath2Quality/1
  LM_EMLFntPathQualityCalc/3(LM_EMLFntPath3Quality) -> LM_EMLFntPath3Quality/1
  LM_EMLFntPathParCalc/1(LM_EMLFntPath1P) -> LM_EMLFntPath1P/1
  LM_EMLFntPathParCalc/2(LM_EMLFntPath2P) -> LM_EMLFntPath2P/1
  LM_EMLFntPathParCalc/3(LM_EMLFntPath3P) -> LM_EMLFntPath3P/1
  LM_DrivInWLType/1 -> LM_EML_C0/1(LM_DrivInWLType)
  LM_EML_C0/1(LM_EMLLLC0) -> LM_EMLLLC0/1
  LM_EML_C0/2(LM_EMLLRC0) -> LM_EMLLRC0/1
  LM_EML_C0/3(LM_EMLRLC0) -> LM_EMLRLC0/1
  LM_EML_C0/4(LM_EMLRRC0) -> LM_EMLRRC0/1
  kapTraj/1 -> LM_EMLKapAdjVal/1(kapTraj)
  DIR_TurnLeftValid/1 -> LM_EMLKapAdjVal/2(DIR_TurnLeftValid)
  DIR_TurnRightValid/1 -> LM_EMLKapAdjVal/3(DIR_TurnRightValid)
